simulink model "TestHiTechnicPrototypeSensor"  (Simulink 6.4)
settings: Solver=FixedStepDiscrete  SolverMode=SingleTasking  StartTime=0  StopTime=10  FixedStep=0.001  RelTol=1e-3
libraries: ecrobot_nxt_lib x4
settings Model: Creator=tchikama  LastModifiedBy=tchikama  ProdHWDeviceType=ARM7
settings DataIOCC: SaveOutput=off  SignalLogging=off  SaveTime=off
settings OptimizationCC: InlineParams=on  InlineInvariantSignals=on  RollThreshold=2  StateBitsets=on  DataBitsets=on  UseTempVars=on  InitFltsAndDblsToZero=off  NoFixptDivByZeroProtection=on  EfficientFloat2IntCast=on  OptimizeModelRefInitCode=on  LifeSpan=1
settings DebuggingCC: ConsistencyChecking=warning  SignalInfNanChecking=warning  ReadBeforeWriteMsg=DisableAll  WriteAfterWriteMsg=DisableAll  WriteAfterReadMsg=DisableAll  AlgebraicLoopMsg=error  CheckExecutionContextPreStartOutputMsg=on  CheckExecutionContextRuntimeOutputMsg=on  SolverPrmCheckMsg=none  SingleTaskRateTransMsg=warning  TasksWithSamePriorityMsg=none  IntegerOverflowMsg=error  ParameterPrecisionLossMsg=none  UnconnectedInputMsg=error  UnconnectedOutputMsg=error  UnconnectedLineMsg=error  UniqueDataStoreMsg=error  BusObjectLabelMismatch=error  RootOutportRequireBusObject=error  ModelReferenceIOMsg=warning  ModelReferenceVersionMismatchMessage=warning  ModelReferenceIOMismatchMessage=warning
settings HardwareCC: ProdIntDivRoundTo=Zero  ProdEndianess=LittleEndian  ProdHWDeviceType=ARM7  TargetHWDeviceType=32-bit Generic
settings ModelReferenceCC: ModelReferenceNumInstancesAllowed=Single
settings RTWCC: SystemTargetFile=ert.tlc  GenCodeOnly=on  GenerateMakefile=off  TemplateMakefile=ert_default_tmf  Description=Real-Time Workshop Embedded Coder (no auto configuration)  GenerateReport=on  RTWVerbose=off  ProcessScript=ert_make_rtw_hook  IncludeHyperlinkInReport=on  LaunchReport=on
settings CodeAppCC: ForceParamTrailComments=on  IgnoreCustomStorageClasses=off  SFDataObjDesc=on  PrefixModelToSubsysFcnNames=off  CustomSymbolStrGlobalVar=rt$N$M  CustomSymbolStrType=$N$M  CustomSymbolStrFcn=$N$M$F  CustomSymbolStrMacro=$N$M  InsertBlockDesc=on
settings ERTTargetCC: TargetFcnLib=ansi_tfl_tmw.mat  GenFloatMathFcnCalls=GNU  IncludeMdlTerminateFcn=off  SuppressErrorStatus=on  IncludeERTFirstTime=on  SupportAbsoluteTime=off  SupportNonFinite=off  SupportComplex=off  PurelyIntegerCode=on  InlinedParameterPlacement=NonHierarchical  RootIOFormat=Structure reference  ERTCustomFileTemplate=example_file_process.tlc  InitialValueSource=Model

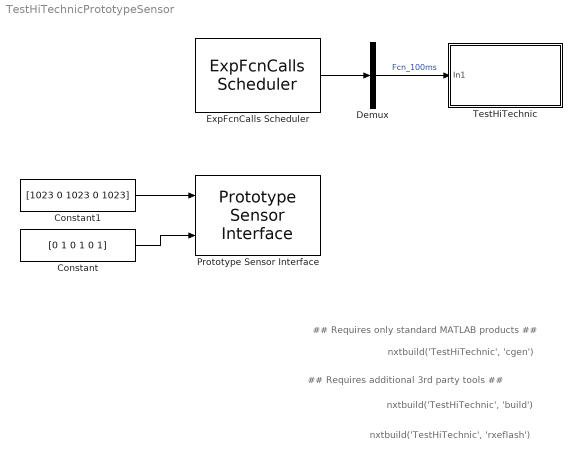
== system TestHiTechnicPrototypeSensor ==
  note: nxtbuild('TestHiTechnic', 'build')
  note: nxtbuild('TestHiTechnic', 'rxeflash')
  note: nxtbuild('TestHiTechnic', 'cgen')
  note: ## Requires only standard MATLAB products ##
  note: ## Requires additional 3rd party tools ##
  Constant : Constant  Value=[0 1 0 1 0 1]  OutDataType=sfix(16)  ConRadixGroup=Use specified scaling  OutScaling=2^0  SampleTime=inf  FramePeriod=inf
  Constant1 : Constant  Value=[1023 0 1023 0 1023]  OutDataType=sfix(16)  ConRadixGroup=Use specified scaling  OutScaling=2^0  SampleTime=inf  FramePeriod=inf
  Demux : Demux  Outputs=1
  ExpFcnCalls Scheduler : ecrobot_nxt_lib/ExpFcnCalls Scheduler  fcname='Fcn_100ms'  fctrigger=[100]  ts=0.001  platform=OSEK  stacksize=[512]  bd_mode=Slave
  Prototype Sensor Interface : ecrobot_nxt_lib/Prototype Sensor Interface  SystemSampleTime=-1  ip=S1
  TestHiTechnic : Subsystem
  wires:
  ExpFcnCalls Scheduler/1 -> Demux/1
  Demux/1 -> TestHiTechnic/1(In1)  "Fcn_100ms"
  Constant1/1 -> Prototype Sensor Interface/1
  Constant/1 -> Prototype Sensor Interface/2

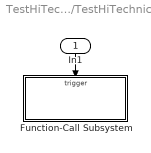
== system TestHiTechnicPrototypeSensor/TestHiTechnic ==
  In1 : Inport  Orientation=down
  Function-Call Subsystem : Subsystem  TreatAsAtomicUnit=on
  wires:
  In1/1 -> Function-Call Subsystem/Trigger

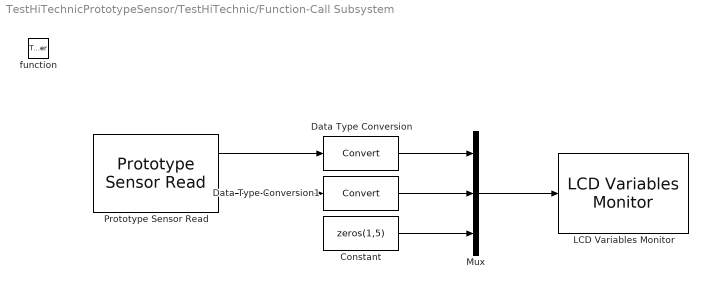
== system TestHiTechnicPrototypeSensor/TestHiTechnic/Function-Call Subsystem ==
  function : TriggerPort  TriggerType=function-call
  Constant : Constant  Value=zeros(1,5)  OutDataTypeMode=int32  OutDataType=sfix(16)  ConRadixGroup=Use specified scaling  OutScaling=2^0  SampleTime=inf  FramePeriod=inf
  Data Type Conversion : DataTypeConversion  OutDataTypeMode=int32
  Data Type Conversion1 : DataTypeConversion  OutDataTypeMode=int32
  LCD Variables Monitor : ecrobot_nxt_lib/LCD Variables Monitor
  Mux : Mux  Inputs=3
  Prototype Sensor Read : ecrobot_nxt_lib/Prototype Sensor Read  ip=S1  sensor_sample_time=100
  wires:
  Data Type Conversion/1 -> Mux/1
  Constant/1 -> Mux/3
  Prototype Sensor Read/1 -> Data Type Conversion/1
  Prototype Sensor Read/2 -> Data Type Conversion1/1
  Data Type Conversion1/1 -> Mux/2
  Mux/1 -> LCD Variables Monitor/1
